simulink subsystem "Autonomously_Navigate_Poses"  (R2023b)
settings: Solver=VariableStepAuto  StartTime=0.0  StopTime=10.0  RelTol=1e-3
undefined symbols (not defined in the file): Spline_Num_Samples, Spline_Stop_Radius
libraries: simulink x3
settings Model: Creator=FIRSTMentor  LastModifiedBy=ander

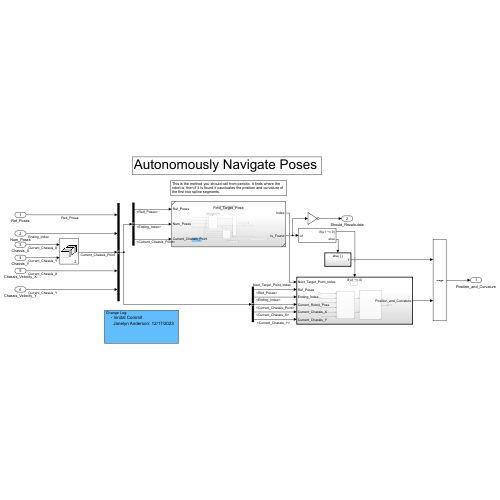
[thumbnail: Simulink's stored preview of the top-level diagram]
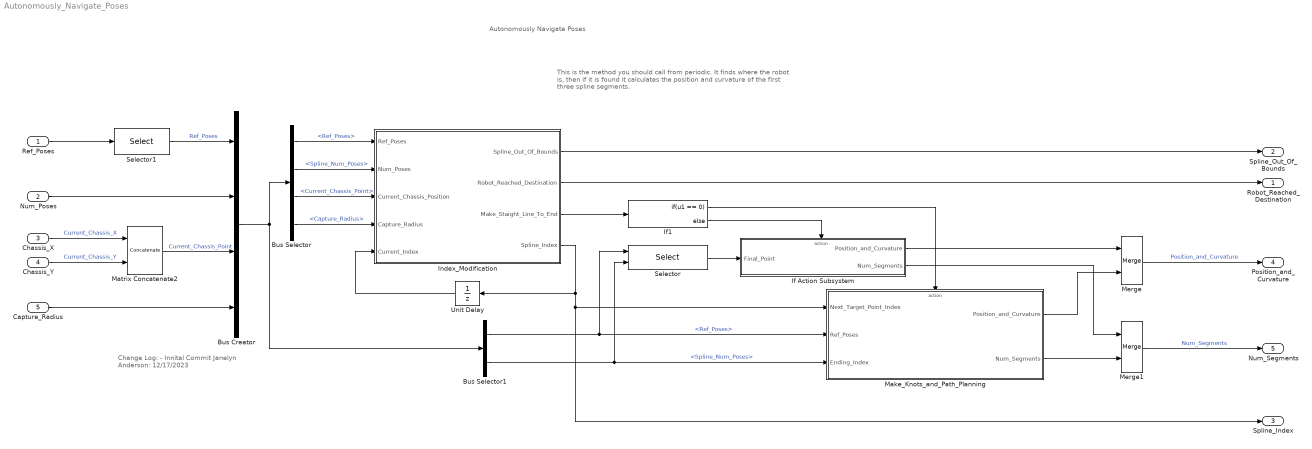
== system Autonomously_Navigate_Poses ==
  note: Autonomously Navigate Poses
  note: This is the method you should call from periodic. It finds where the robot is, then if it is found it calculates the position and curvature of the first three spline segments.
  note: Change Log:
      | - Innital Commit
      | Janelyn Anderson: 12/17/2023
  Ref_Poses : Inport  OutDataTypeStr=double
  Num_Poses : Inport  Port=2  OutDataTypeStr=double  PortDimensions=1
  Chassis_X : Inport  Port=3  OutDataTypeStr=double  PortDimensions=1
  Chassis_Y : Inport  Port=4  OutDataTypeStr=double  PortDimensions=1
  Capture_Radius : Inport  Port=5
  Bus Creator : BusCreator  Inputs=4
  Bus Selector : BusSelector  OutputSignals=Ref_Poses,Spline_Num_Poses,Current_Chassis_Point,Capture_Radius
  Bus Selector1 : BusSelector  OutputSignals=Ref_Poses,Spline_Num_Poses
  If Action Subsystem : Subsystem  TreatAsAtomicUnit=on
  If1 : If  IfExpression=u1 == 0
  Index_Modification : Subsystem
  Make_Knots_and_Path_Planning : Subsystem
  Matrix Concatenate2 : Concatenate  Mode=Multidimensional array  ConcatenateDimension=2
  Merge : Merge
  Merge1 : Merge
  Selector : Selector  NumberOfDimensions=2  InputPortWidth=3  IndexOptions=Index vector (port),Select all  Indices=[1 3],1  OutputSizes=1,1
  Selector1 : Selector  NumberOfDimensions=2  InputPortWidth=3  IndexOptions=Select all,Index vector (dialog)  Indices=[1 3],[1 2]  OutputSizes=1,1
  Unit Delay : UnitDelay  InitialCondition=2  SampleTime=-1  HasFrameUpgradeWarning=on
      settings: AttributesFormatString=IC: %<InitialCondition>
  Robot_Reached_Destination : Outport
  Spline_Out_Of_Bounds : Outport  Port=2
  Spline_Index : Outport  Port=3
  Position_and_Curvature : Outport  Port=4  PortDimensions=[Spline_Num_Samples,3,3]
  Num_Segments : Outport  Port=5
  wires:
  Merge/1 -> Position_and_Curvature/1  "Position_and_Curvature"
  If Action Subsystem/1(Position_and_Curvature) -> Merge/1
  Bus Selector1/1 -> Selector/1, Make_Knots_and_Path_Planning/2(Ref_Poses)  "<Ref_Poses>"
  Bus Selector1/2 -> Make_Knots_and_Path_Planning/3(Ending_Index), Selector/2  "<Spline_Num_Poses>"
  Bus Creator/1 -> Bus Selector1/1, Bus Selector/1
  Num_Poses/1 -> Bus Creator/2
  Make_Knots_and_Path_Planning/1(Position_and_Curvature) -> Merge/2
  Ref_Poses/1 -> Selector1/1
  Matrix Concatenate2/1 -> Bus Creator/3  "Current_Chassis_Point"
  Chassis_Y/1 -> Matrix Concatenate2/2  "Current_Chassis_Y"
  Chassis_X/1 -> Matrix Concatenate2/1  "Current_Chassis_X"
  Make_Knots_and_Path_Planning/2(Num_Segments) -> Merge1/2
  Merge1/1 -> Num_Segments/1  "Num_Segments"
  If Action Subsystem/2(Num_Segments) -> Merge1/1
  Selector/1 -> If Action Subsystem/1(Final_Point)
  Index_Modification/4(Spline_Index) -> Make_Knots_and_Path_Planning/1(Next_Target_Point_Index), Spline_Index/1, Unit Delay/1
  Unit Delay/1 -> Index_Modification/5(Current_Index)
  Index_Modification/3(Make_Staight_Line_To_End) -> If1/1
  If1/1 -> Make_Knots_and_Path_Planning/Action
  If1/2 -> If Action Subsystem/Action
  Index_Modification/2(Robot_Reached_Destination) -> Robot_Reached_Destination/1
  Index_Modification/1(Spline_Out_Of_Bounds) -> Spline_Out_Of_Bounds/1
  Bus Selector/1 -> Index_Modification/1(Ref_Poses)  "<Ref_Poses>"
  Bus Selector/2 -> Index_Modification/2(Num_Poses)  "<Spline_Num_Poses>"
  Bus Selector/3 -> Index_Modification/3(Current_Chassis_Position)  "<Current_Chassis_Point>"
  Selector1/1 -> Bus Creator/1  "Ref_Poses"
  Capture_Radius/1 -> Bus Creator/4
  Bus Selector/4 -> Index_Modification/4(Capture_Radius)  "<Capture_Radius>"

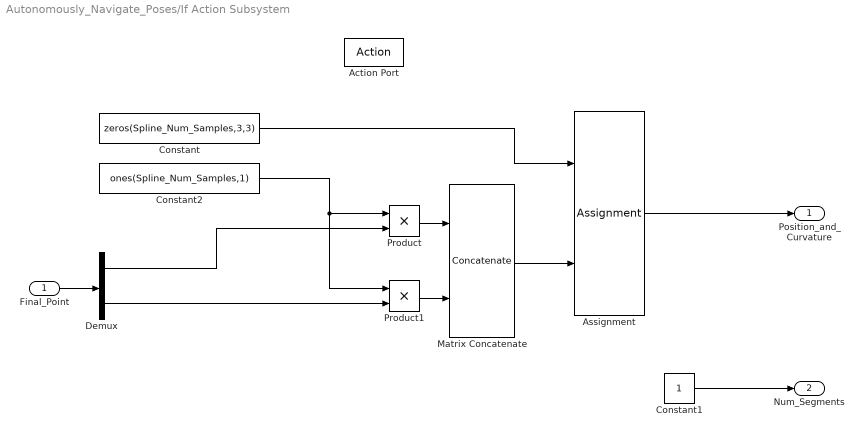
== system Autonomously_Navigate_Poses/If Action Subsystem ==
  Final_Point : Inport
  Action Port : ActionPort  InitializeStates=reset
  Assignment : Assignment  NumberOfDimensions=3  DiagnosticForDimensions=Warning  IndexOptions=Assign all,Starting index (dialog),Index vector (dialog)  Indices=1,1,1  OutputSizes=1,1,1
  Constant : Constant  Value=zeros(Spline_Num_Samples,3,3)
  Constant1 : Constant  OutDataTypeStr=int32
  Constant2 : Constant  Value=ones(Spline_Num_Samples,1)  VectorParams1D=off  OutDataTypeStr=int32
  Demux : Demux  Outputs=2
  Matrix Concatenate : Concatenate  Mode=Multidimensional array  ConcatenateDimension=2
  Product : Product
  Product1 : Product
  Position_and_Curvature : Outport
  Num_Segments : Outport  Port=2
  wires:
  Demux/2 -> Product1/2
  Demux/1 -> Product/2
  Constant2/1 -> Product/1, Product1/1
  Product1/1 -> Matrix Concatenate/2
  Product/1 -> Matrix Concatenate/1
  Final_Point/1 -> Demux/1
  Matrix Concatenate/1 -> Assignment/2
  Assignment/1 -> Position_and_Curvature/1
  Constant1/1 -> Num_Segments/1
  Constant/1 -> Assignment/1

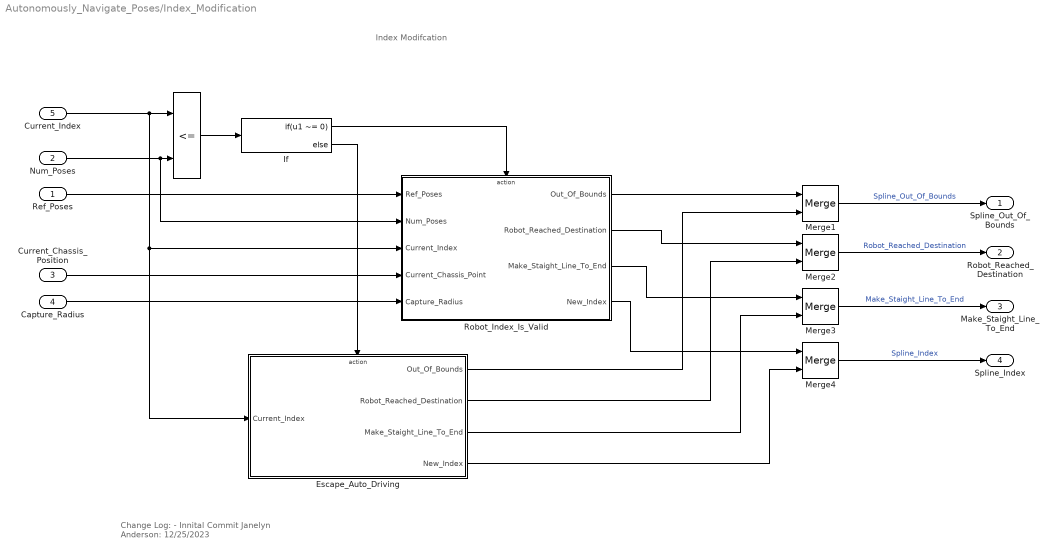
== system Autonomously_Navigate_Poses/Index_Modification ==
  note: Change Log:
      | - Innital Commit
      | Janelyn Anderson: 12/25/2023
  note: Index Modifcation
  Ref_Poses : Inport
  Num_Poses : Inport  Port=2
  Current_Chassis_Position : Inport  Port=3
  Capture_Radius : Inport  Port=4
  Current_Index : Inport  Port=5
  " " : RelationalOperator  Operator=<=  OutDataTypeStr=boolean  RndMeth=Simplest  InputSameDT=off
  Escape_Auto_Driving : Subsystem  TreatAsAtomicUnit=on
  If : If  IfExpression=u1 ~= 0
  Merge{1..4} (4 alike) : Merge
  Robot_Index_Is_Valid : Subsystem  TreatAsAtomicUnit=on
  Spline_Out_Of_Bounds : Outport
  Robot_Reached_Destination : Outport  Port=2
  Make_Staight_Line_To_End : Outport  Port=3
  Spline_Index : Outport  Port=4
  wires:
  Capture_Radius/1 -> Robot_Index_Is_Valid/5(Capture_Radius)
  Current_Chassis_Position/1 -> Robot_Index_Is_Valid/4(Current_Chassis_Point)
  Ref_Poses/1 -> Robot_Index_Is_Valid/1(Ref_Poses)
  Escape_Auto_Driving/4(New_Index) -> Merge4/2
  Escape_Auto_Driving/3(Make_Staight_Line_To_End) -> Merge3/2
  Escape_Auto_Driving/2(Robot_Reached_Destination) -> Merge2/2
  Escape_Auto_Driving/1(Out_Of_Bounds) -> Merge1/2
  Robot_Index_Is_Valid/4(New_Index) -> Merge4/1
  Robot_Index_Is_Valid/3(Make_Staight_Line_To_End) -> Merge3/1
  Robot_Index_Is_Valid/2(Robot_Reached_Destination) -> Merge2/1
  Robot_Index_Is_Valid/1(Out_Of_Bounds) -> Merge1/1
  Merge1/1 -> Spline_Out_Of_Bounds/1  "Spline_Out_Of_Bounds"
  Merge2/1 -> Robot_Reached_Destination/1  "Robot_Reached_Destination"
  Merge3/1 -> Make_Staight_Line_To_End/1  "Make_Staight_Line_To_End"
  Merge4/1 -> Spline_Index/1  "Spline_Index"
  If/2 -> Escape_Auto_Driving/Action
  If/1 -> Robot_Index_Is_Valid/Action
  " "/1 -> If/1
  Num_Poses/1 -> " "/2, Robot_Index_Is_Valid/2(Num_Poses)
  Current_Index/1 -> " "/1, Robot_Index_Is_Valid/3(Current_Index), Escape_Auto_Driving/1(Current_Index)

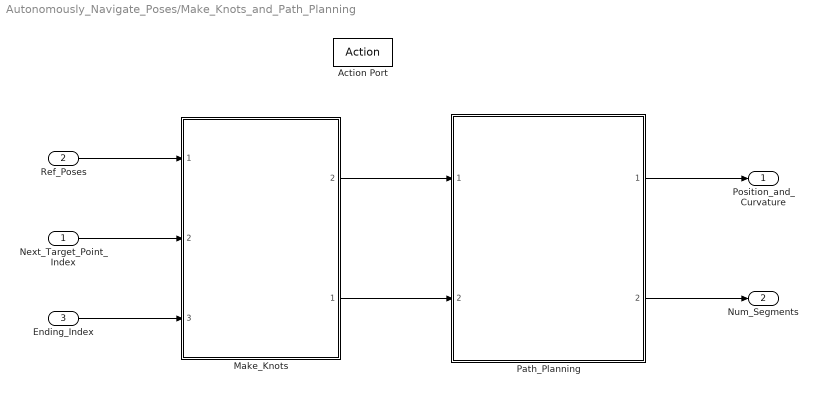
== system Autonomously_Navigate_Poses/Make_Knots_and_Path_Planning ==
  Next_Target_Point_Index : Inport
  Ref_Poses : Inport  Port=2
  Ending_Index : Inport  Port=3
  Action Port : ActionPort  InitializeStates=reset  PropagateVarSize=During execution
  Make_Knots : Subsystem  ReferencedSubsystem=Make_Knots
      settings: PortSchema="{\"entries\":[{\"content\":{\"sides\":[{\"content\":{\"connectorIds\":[\"In1\",\"In2\",\"In3\"]},\"type\":\"ConnectorPlacement.EquallySpacedRectSide\",\"uuid\":\"ef14d2d2-5e89-4728-9616-9c294df62418\"},{\"content\":{\"connectorIds\":[\"Out2\",\"Out1\"],\"side\":\"RIGHT\"},\"type\":\"ConnectorPlacement.EquallySpacedRectSide\",\"uuid\":\"1981533b-8fa5-400f-9c0f-906ffb1c32b1\"},{\"content\":{\"side\":\"TOP\"},\"type\":\"ConnectorPlacement.EquallySpacedRectSide\",\"uuid\":\"42309c84-0d64-4907-9713-531b28904217\"}]},\"type\":\"ConnectorPlacement.EquallySpacedConnector\",\"uuid\":\"4fb29ac0-3c61-4bdf-ba6b-9fa70e8815da\"}],\"packageUris\":[\"http://schema.mathworks.com/mf0/Connector/R2020b\"],\"version\":\"1.0\"}"
  Path_Planning : Subsystem  ReferencedSubsystem=Path_Planning
  Position_and_Curvature : Outport  PortDimensions=[Spline_Num_Samples,3,3]
  Num_Segments : Outport  Port=2
  wires:
  Path_Planning/2 -> Num_Segments/1
  Ref_Poses/1 -> Make_Knots/1
  Next_Target_Point_Index/1 -> Make_Knots/2
  Ending_Index/1 -> Make_Knots/3
  Make_Knots/2 -> Path_Planning/1
  Make_Knots/1 -> Path_Planning/2
  Path_Planning/1 -> Position_and_Curvature/1

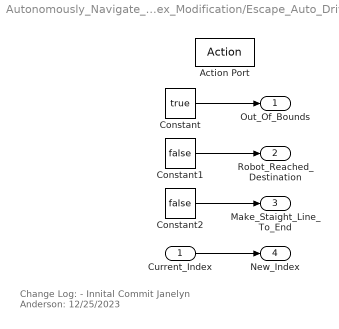
== system Autonomously_Navigate_Poses/Index_Modification/Escape_Auto_Driving ==
  note: Change Log:
      | - Innital Commit
      | Janelyn Anderson: 12/25/2023
  Current_Index : Inport
  Action Port : ActionPort  InitializeStates=reset
  Constant : Constant  Value=true
  Constant1 : Constant  Value=false
  Constant2 : Constant  Value=false
  Out_Of_Bounds : Outport
  Robot_Reached_Destination : Outport  Port=2
  Make_Staight_Line_To_End : Outport  Port=3
  New_Index : Outport  Port=4
  wires:
  Constant2/1 -> Make_Staight_Line_To_End/1
  Constant1/1 -> Robot_Reached_Destination/1
  Constant/1 -> Out_Of_Bounds/1
  Current_Index/1 -> New_Index/1

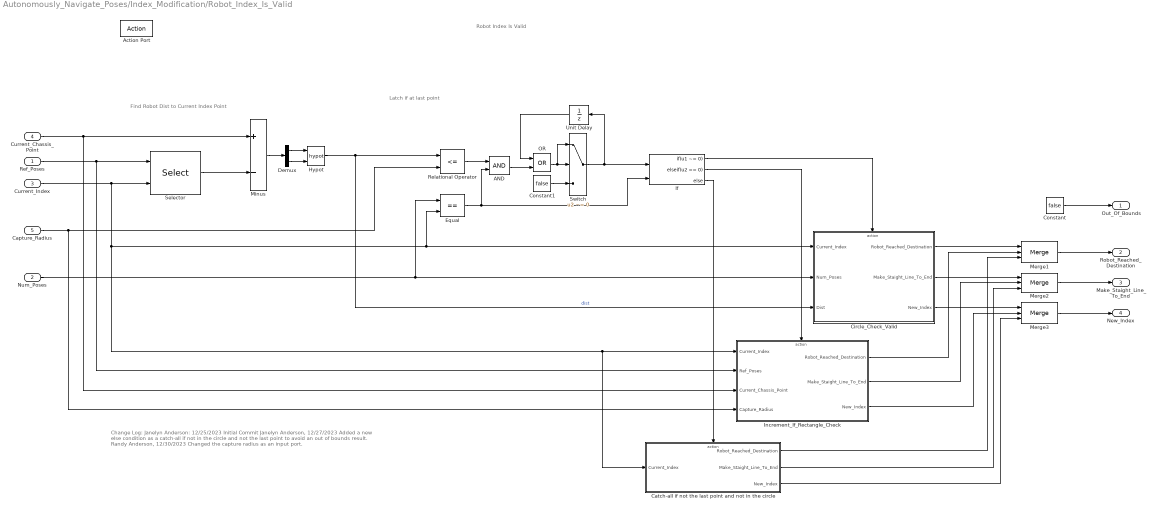
== system Autonomously_Navigate_Poses/Index_Modification/Robot_Index_Is_Valid ==
  note: Change Log:
      | Janelyn Anderson: 12/25/2023
      | Initial Commit
      | Janelyn Anderson, 12/27/2023
      | Added a new else condition as a catch-all if not in the circle and not the last point to avoid an out of bounds result.
      | Randy Anderson, 12/30/2023
      | Changed the capture radius as an input port.
  note: Robot Index Is Valid
  note: Latch if at last point
  note: Find Robot Dist to Current Index Point
  Ref_Poses : Inport
  Num_Poses : Inport  Port=2
  Current_Index : Inport  Port=3
  Current_Chassis_Point : Inport  Port=4
  Capture_Radius : Inport  Port=5
  Action Port : ActionPort  InitializeStates=reset
  AND : Logic  AllPortsSameDT=off  OutDataTypeStr=boolean
  Catch-all if not the last point and not in the circle : Subsystem  TreatAsAtomicUnit=on
  Circle_Check_Valid : Subsystem  TreatAsAtomicUnit=on
  Constant : Constant  Value=false
  Constant1 : Constant  Value=false
  Demux : Demux  Outputs=2
  Equal : RelationalOperator  Operator===  OutDataTypeStr=boolean  RndMeth=Simplest  InputSameDT=off
  Hypot : Math  Operator=hypot
  If : If  NumInputs=2  IfExpression=u1 ~= 0  ElseIfExpressions=u2 == 0
  Increment_If_Rectangle_Check : Subsystem  TreatAsAtomicUnit=on
  Merge1 : Merge  Inputs=3
  Merge2 : Merge  Inputs=3
  Merge3 : Merge  Inputs=3
  Minus : Sum  Inputs=+-
  OR : Logic  Operator=OR  AllPortsSameDT=off  OutDataTypeStr=boolean
  Relational Operator : RelationalOperator  Operator=<=  OutDataTypeStr=boolean  RndMeth=Simplest  InputSameDT=off
  Selector : Selector  NumberOfDimensions=2  InputPortWidth=3  IndexOptions=Index vector (port),Select all  Indices=[1 3],1  OutputSizes=1,1
  Switch : Switch  Criteria=u2 ~= 0  SaturateOnIntegerOverflow=off  InputSameDT=off
  Unit Delay : UnitDelay  SampleTime=-1  HasFrameUpgradeWarning=on
  Out_Of_Bounds : Outport
  Robot_Reached_Destination : Outport  Port=2
  Make_Staight_Line_To_End : Outport  Port=3
  New_Index : Outport  Port=4
  wires:
  Capture_Radius/1 -> Increment_If_Rectangle_Check/4(Capture_Radius), Relational Operator/2
  Catch-all if not the last point and not in the circle/3(New_Index) -> Merge3/3
  Catch-all if not the last point and not in the circle/2(Make_Staight_Line_To_End) -> Merge2/3
  Catch-all if not the last point and not in the circle/1(Robot_Reached_Destination) -> Merge1/3
  If/3 -> Catch-all if not the last point and not in the circle/Action
  Constant1/1 -> Switch/3
  Unit Delay/1 -> OR/1
  Switch/1 -> If/1, Unit Delay/1
  OR/1 -> Switch/2, Switch/1
  AND/1 -> OR/2
  Equal/1 -> If/2, AND/2
  Relational Operator/1 -> AND/1
  Num_Poses/1 -> Circle_Check_Valid/2(Num_Poses), Equal/1
  Increment_If_Rectangle_Check/3(New_Index) -> Merge3/2
  Increment_If_Rectangle_Check/2(Make_Staight_Line_To_End) -> Merge2/2
  Increment_If_Rectangle_Check/1(Robot_Reached_Destination) -> Merge1/2
  Circle_Check_Valid/3(New_Index) -> Merge3/1
  Circle_Check_Valid/2(Make_Staight_Line_To_End) -> Merge2/1
  Circle_Check_Valid/1(Robot_Reached_Destination) -> Merge1/1
  Merge3/1 -> New_Index/1
  Merge2/1 -> Make_Staight_Line_To_End/1
  Merge1/1 -> Robot_Reached_Destination/1
  Constant/1 -> Out_Of_Bounds/1
  If/1 -> Circle_Check_Valid/Action
  If/2 -> Increment_If_Rectangle_Check/Action
  Current_Index/1 -> Selector/2, Circle_Check_Valid/1(Current_Index), Equal/2, Increment_If_Rectangle_Check/1(Current_Index), Catch-all if not the last point and not in the circle/1(Current_Index)
  Hypot/1 -> Circle_Check_Valid/3(Dist), Relational Operator/1  "dist"
  Minus/1 -> Demux/1
  Current_Chassis_Point/1 -> Increment_If_Rectangle_Check/3(Current_Chassis_Point), Minus/1
  Selector/1 -> Minus/2
  Ref_Poses/1 -> Increment_If_Rectangle_Check/2(Ref_Poses), Selector/1
  Demux/2 -> Hypot/2
  Demux/1 -> Hypot/1

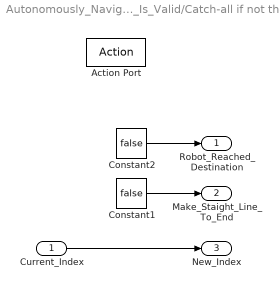
== system Autonomously_Navigate_Poses/Index_Modification/Robot_Index_Is_Valid/Catch-all if not the last point and not in the circle ==
  Current_Index : Inport
  Action Port : ActionPort
  Constant1 : Constant  Value=false
  Constant2 : Constant  Value=false
  Robot_Reached_Destination : Outport
  Make_Staight_Line_To_End : Outport  Port=2
  New_Index : Outport  Port=3
  wires:
  Current_Index/1 -> New_Index/1
  Constant2/1 -> Robot_Reached_Destination/1
  Constant1/1 -> Make_Staight_Line_To_End/1

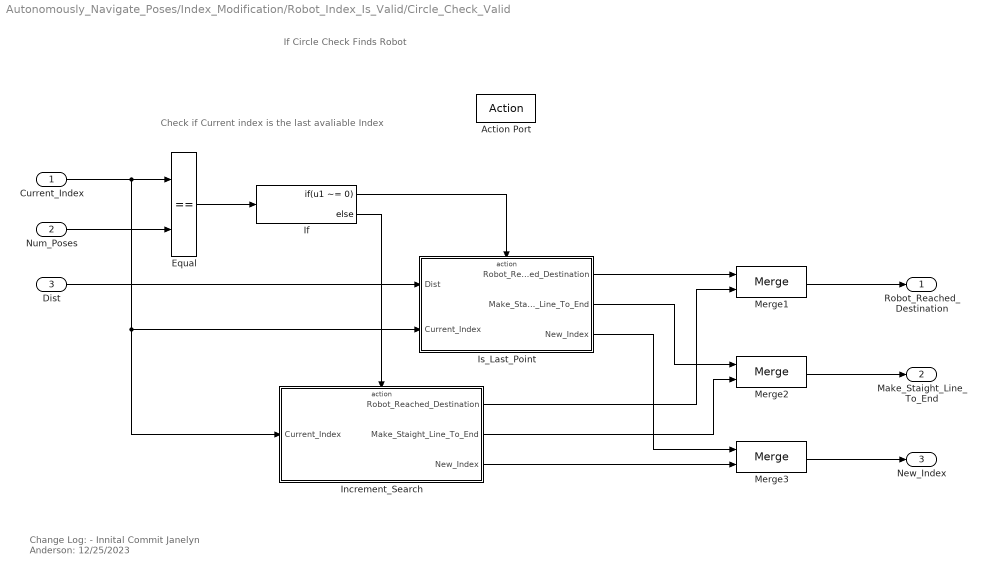
== system Autonomously_Navigate_Poses/Index_Modification/Robot_Index_Is_Valid/Circle_Check_Valid ==
  note: Change Log:
      | - Innital Commit
      | Janelyn Anderson: 12/25/2023
  note: If Circle Check Finds Robot
  note: Check if Current index
      | is the last avaliable Index
  Current_Index : Inport
  Num_Poses : Inport  Port=2
  Dist : Inport  Port=3
  Action Port : ActionPort  InitializeStates=reset
  Equal : RelationalOperator  Operator===  OutDataTypeStr=boolean  RndMeth=Simplest  InputSameDT=off
  If : If  IfExpression=u1 ~= 0
  Increment_Search : Subsystem  TreatAsAtomicUnit=on
  Is_Last_Point : Subsystem  TreatAsAtomicUnit=on
  Merge1 : Merge
  Merge2 : Merge
  Merge3 : Merge
  Robot_Reached_Destination : Outport
  Make_Staight_Line_To_End : Outport  Port=2
  New_Index : Outport  Port=3
  wires:
  Is_Last_Point/3(New_Index) -> Merge3/1
  Is_Last_Point/2(Make_Staight_Line_To_End) -> Merge2/1
  Is_Last_Point/1(Robot_Reached_Destination) -> Merge1/1
  Increment_Search/1(Robot_Reached_Destination) -> Merge1/2
  Increment_Search/2(Make_Staight_Line_To_End) -> Merge2/2
  Increment_Search/3(New_Index) -> Merge3/2
  Merge2/1 -> Make_Staight_Line_To_End/1
  Merge3/1 -> New_Index/1
  Merge1/1 -> Robot_Reached_Destination/1
  Dist/1 -> Is_Last_Point/1(Dist)
  If/1 -> Is_Last_Point/Action
  If/2 -> Increment_Search/Action
  Equal/1 -> If/1
  Num_Poses/1 -> Equal/2
  Current_Index/1 -> Increment_Search/1(Current_Index), Is_Last_Point/2(Current_Index), Equal/1

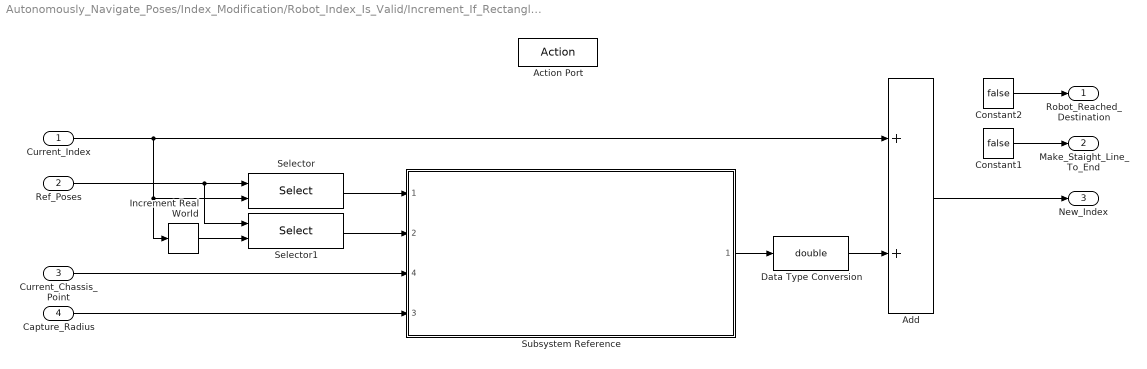
== system Autonomously_Navigate_Poses/Index_Modification/Robot_Index_Is_Valid/Increment_If_Rectangle_Check ==
  Current_Index : Inport
  Ref_Poses : Inport  Port=2
  Current_Chassis_Point : Inport  Port=3
  Capture_Radius : Inport  Port=4
  Action Port : ActionPort  InitializeStates=reset
  Add : Sum
  Constant1 : Constant  Value=false
  Constant2 : Constant  Value=false
  Data Type Conversion : DataTypeConversion  OutDataTypeStr=double  SaturateOnIntegerOverflow=off  RndMeth=Floor
  Increment Real World : simulink/Additional Math & Discrete/Additional Math: Increment - Decrement/Increment Real World
  Selector : Selector  NumberOfDimensions=2  InputPortWidth=3  IndexOptions=Index vector (port),Select all  Indices=[1 3],1  OutputSizes=1,1
  Selector1 : Selector  NumberOfDimensions=2  InputPortWidth=3  IndexOptions=Index vector (port),Select all  Indices=[1 3],1  OutputSizes=1,1
  Subsystem Reference : Subsystem  ReferencedSubsystem=Bandwidth_Check_Between_Two_Points
      settings: PortSchema="{\"entries\":[{\"content\":{\"sides\":[{\"content\":{\"connectorIds\":[\"In1\",\"In2\",\"In4\",\"In3\"]},\"type\":\"ConnectorPlacement.EquallySpacedRectSide\",\"uuid\":\"ceb776b8-c050-4a98-93b2-29d0e514edc7\"},{\"content\":{\"connectorIds\":[\"Out1\"],\"side\":\"RIGHT\"},\"type\":\"ConnectorPlacement.EquallySpacedRectSide\",\"uuid\":\"6b0bd286-7e09-4672-ae75-d20305541db2\"},{\"content\":{\"side\":\"TOP\"},\"type\":\"ConnectorPlacement.EquallySpacedRectSide\",\"uuid\":\"2a1e7e93-e406-49f3-8e81-1c2419e85ee2\"}]},\"type\":\"ConnectorPlacement.EquallySpacedConnector\",\"uuid\":\"a612ddb7-ae02-43ab-a30c-20f014ad7d06\"}],\"packageUris\":[\"http://schema.mathworks.com/mf0/Connector/R2020b\"],\"version\":\"1.0\"}"
  Robot_Reached_Destination : Outport
  Make_Staight_Line_To_End : Outport  Port=2
  New_Index : Outport  Port=3
  wires:
  Capture_Radius/1 -> Subsystem Reference/3
  Constant2/1 -> Robot_Reached_Destination/1
  Constant1/1 -> Make_Staight_Line_To_End/1
  Ref_Poses/1 -> Selector1/1, Selector/1
  Increment Real World/1 -> Selector1/2
  Selector1/1 -> Subsystem Reference/2
  Selector/1 -> Subsystem Reference/1
  Current_Chassis_Point/1 -> Subsystem Reference/4
  Add/1 -> New_Index/1
  Current_Index/1 -> Increment Real World/1, Selector/2, Add/1
  Data Type Conversion/1 -> Add/2
  Subsystem Reference/1 -> Data Type Conversion/1

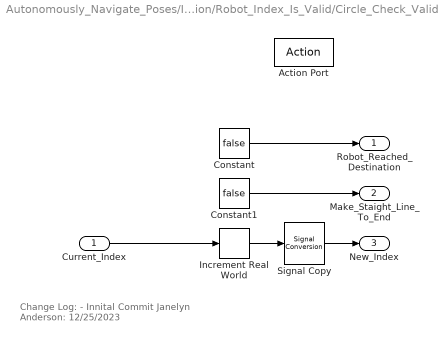
== system Autonomously_Navigate_Poses/Index_Modification/Robot_Index_Is_Valid/Circle_Check_Valid/Increment_Search ==
  note: Change Log:
      | - Innital Commit
      | Janelyn Anderson: 12/25/2023
  Current_Index : Inport
  Action Port : ActionPort  InitializeStates=reset
  Constant : Constant  Value=false
  Constant1 : Constant  Value=false
  Increment Real World : simulink/Additional Math & Discrete/Additional Math: Increment - Decrement/Increment Real World
  Signal Copy : SignalConversion  OverrideOpt=off
  Robot_Reached_Destination : Outport
  Make_Staight_Line_To_End : Outport  Port=2
  New_Index : Outport  Port=3
  wires:
  Signal Copy/1 -> New_Index/1
  Constant/1 -> Robot_Reached_Destination/1
  Constant1/1 -> Make_Staight_Line_To_End/1
  Increment Real World/1 -> Signal Copy/1
  Current_Index/1 -> Increment Real World/1

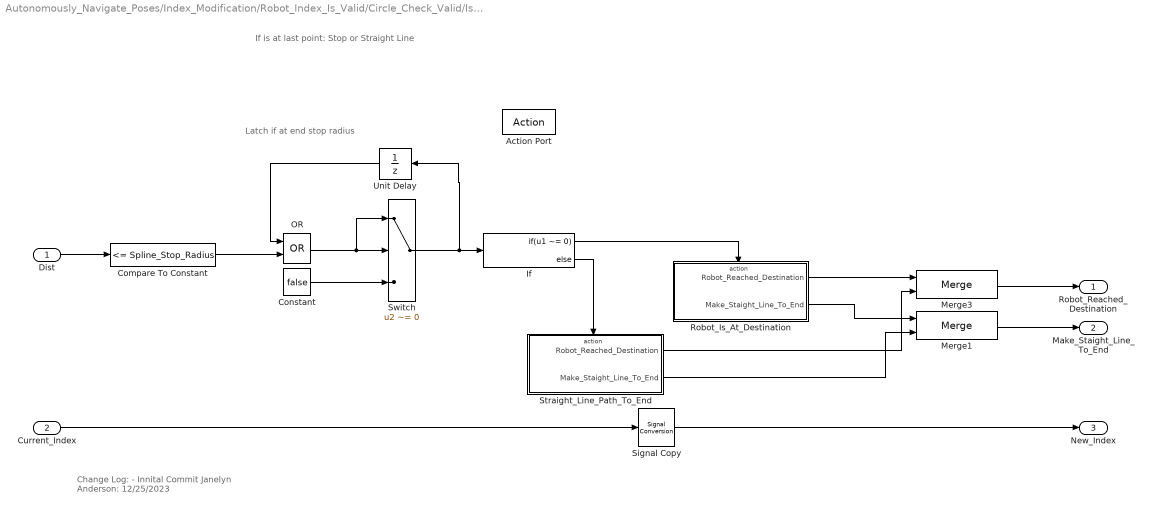
== system Autonomously_Navigate_Poses/Index_Modification/Robot_Index_Is_Valid/Circle_Check_Valid/Is_Last_Point ==
  note: Change Log:
      | - Innital Commit
      | Janelyn Anderson: 12/25/2023
  note: If is at last point: Stop or Straight Line
  note: Latch if at end stop radius
  Dist : Inport
  Current_Index : Inport  Port=2
  Action Port : ActionPort  InitializeStates=reset
  Compare To Constant : simulink/Logic and Bit Operations/Compare To Constant  relop=<=  const=Spline_Stop_Radius  OutDataTypeStr=boolean
  Constant : Constant  Value=false
  If : If  IfExpression=u1 ~= 0
  Merge1 : Merge
  Merge3 : Merge
  OR : Logic  Operator=OR  AllPortsSameDT=off  OutDataTypeStr=boolean
  Robot_Is_At_Destination : Subsystem  TreatAsAtomicUnit=on
  Signal Copy : SignalConversion  OverrideOpt=off
  Straight_Line_Path_To_End : Subsystem  TreatAsAtomicUnit=on
  Switch : Switch  Criteria=u2 ~= 0  SaturateOnIntegerOverflow=off  InputSameDT=off
  Unit Delay : UnitDelay  SampleTime=-1  HasFrameUpgradeWarning=on
  Robot_Reached_Destination : Outport
  Make_Staight_Line_To_End : Outport  Port=2
  New_Index : Outport  Port=3
  wires:
  Unit Delay/1 -> OR/1
  Constant/1 -> Switch/3
  OR/1 -> Switch/2, Switch/1
  Compare To Constant/1 -> OR/2
  Switch/1 -> Unit Delay/1, If/1
  Signal Copy/1 -> New_Index/1
  Merge3/1 -> Robot_Reached_Destination/1
  Merge1/1 -> Make_Staight_Line_To_End/1
  Straight_Line_Path_To_End/2(Make_Staight_Line_To_End) -> Merge1/2
  Robot_Is_At_Destination/2(Make_Staight_Line_To_End) -> Merge1/1
  Straight_Line_Path_To_End/1(Robot_Reached_Destination) -> Merge3/2
  Robot_Is_At_Destination/1(Robot_Reached_Destination) -> Merge3/1
  Current_Index/1 -> Signal Copy/1
  Dist/1 -> Compare To Constant/1
  If/2 -> Straight_Line_Path_To_End/Action
  If/1 -> Robot_Is_At_Destination/Action

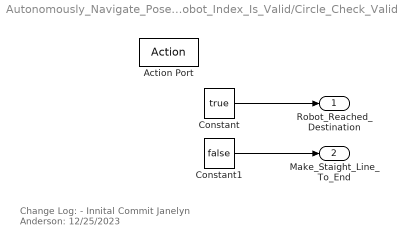
== system Autonomously_Navigate_Poses/Index_Modification/Robot_Index_Is_Valid/Circle_Check_Valid/Is_Last_Point/Robot_Is_At_Destination ==
  note: Change Log:
      | - Innital Commit
      | Janelyn Anderson: 12/25/2023
  Action Port : ActionPort
  Constant : Constant  Value=true
  Constant1 : Constant  Value=false
  Robot_Reached_Destination : Outport
  Make_Staight_Line_To_End : Outport  Port=2
  wires:
  Constant/1 -> Robot_Reached_Destination/1
  Constant1/1 -> Make_Staight_Line_To_End/1

== system Autonomously_Navigate_Poses/Index_Modification/Robot_Index_Is_Valid/Circle_Check_Valid/Is_Last_Point/Straight_Line_Path_To_End ==
  note: Change Log:
      | - Innital Commit
      | Janelyn Anderson: 12/25/2023
  Action Port : ActionPort
  Constant : Constant  Value=false
  Constant1 : Constant  Value=true
  Robot_Reached_Destination : Outport
  Make_Staight_Line_To_End : Outport  Port=2
  wires:
  Constant1/1 -> Make_Staight_Line_To_End/1
  Constant/1 -> Robot_Reached_Destination/1
